simulink model "com_detect_red_circle"  (R2016b)
settings: Solver=VariableStepAuto  StartTime=0.0  StopTime=inf  RelTol=1e-3
values from neighbouring files (symbols this model uses):
  hmax = inrange.h_max_r    [computer_detectTrafficLight.m]    (also in getColorPX.m = h)
  hmin = inrange.h_min_r    [computer_detectTrafficLight.m]    (also in getColorPX.m = h)
  smax = inrange.s_max_r    [computer_detectTrafficLight.m]    (also in getColorPX.m = s)
  smin = inrange.s_min_r    [computer_detectTrafficLight.m]    (also in getColorPX.m = s)
  vmax = inrange.v_max_r    [computer_detectTrafficLight.m]    (also in getColorPX.m = v)
  vmin = inrange.v_min_r    [computer_detectTrafficLight.m]    (also in getColorPX.m = v)
undefined symbols (not defined in the file or in its folder): gray, Rec, SDTV, strel
libraries: etargetslib x15, dspnetwork x15, visionconversions x5, visiongeotforms x3, visionmorphops x2, visiontextngfix x1
settings Model: Creator=zeabus  LastModifiedBy=zeabus

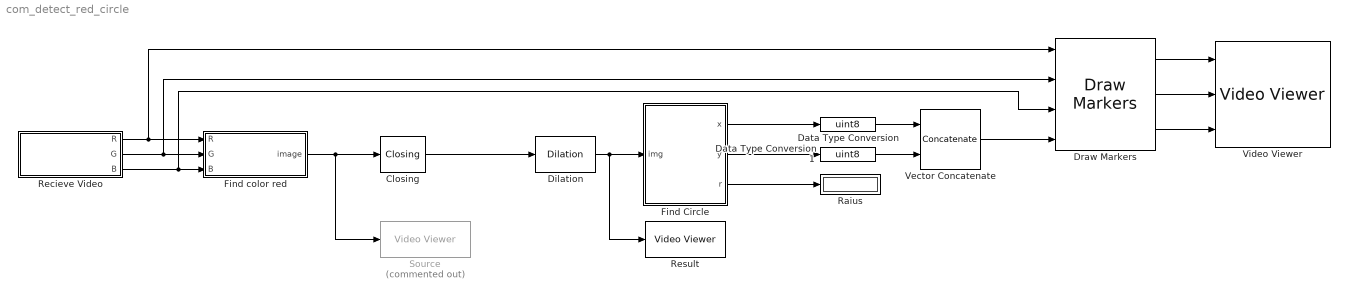
== system com_detect_red_circle ==
  Closing : visionmorphops/Closing  nhoodsrc=Specify via dialog  strel=strel('line', 10, 45)
  Data Type Conversion : DataTypeConversion  OutDataTypeStr=uint8
  Data Type Conversion1 : DataTypeConversion  OutDataTypeStr=uint8
  Dilation : visionmorphops/Dilation  nhoodsrc=Specify via dialog  strel=[40 40 40; 40 40 40; 40 40 40]
  Draw Markers : visiontextngfix/Draw Markers  shape=Circle  size=20  fill=on  fillClrSource=Specify via dialog  display=User-specified value  intensity=200  color=[255 255 0]  opacity=0.6  viewport=Entire image  antialiasing=off  inType=Obsolete  imagePorts=Separate color signals  prodOutputMode=Binary point scaling  prodOutputWordLength=32  prodOutputFracLength=14  memoryMode=Specify word length  memoryWordLength=16  memoryFracLength=14  roundingMode=Floor  overflowMode=off
  Find Circle : MATLAB Function  TreatAsAtomicUnit=on
  Find color red : Subsystem
  Raius : Display
  Recieve Video : Subsystem
  Result : VideoViewer  FigPos=[-15 1005 811 384]
  Source : VideoViewer  Commented=on  colormapValue=gray(256)  FigPos=[-22 597 811 384]
  Vector Concatenate : Concatenate  Mode=Multidimensional array
  Video Viewer : VideoViewer  imagePorts=separate color signals  FigPos=[1334 859 660 461]
  wires:
  Draw Markers/1 -> Video Viewer/1
  Draw Markers/2 -> Video Viewer/2
  Draw Markers/3 -> Video Viewer/3
  Find Circle/1(x) -> Data Type Conversion/1
  Find Circle/2(y) -> Data Type Conversion1/1
  Vector Concatenate/1 -> Draw Markers/4
  Data Type Conversion/1 -> Vector Concatenate/1
  Data Type Conversion1/1 -> Vector Concatenate/2
  Find color red/1(image) -> Source/1, Closing/1
  Dilation/1 -> Result/1, Find Circle/1(img)
  Find Circle/3(r) -> Raius/1
  Closing/1 -> Dilation/1
  Recieve Video/1(R) -> Draw Markers/1, Find color red/1(R)
  Recieve Video/2(G) -> Draw Markers/2, Find color red/2(G)
  Recieve Video/3(B) -> Draw Markers/3, Find color red/3(B)

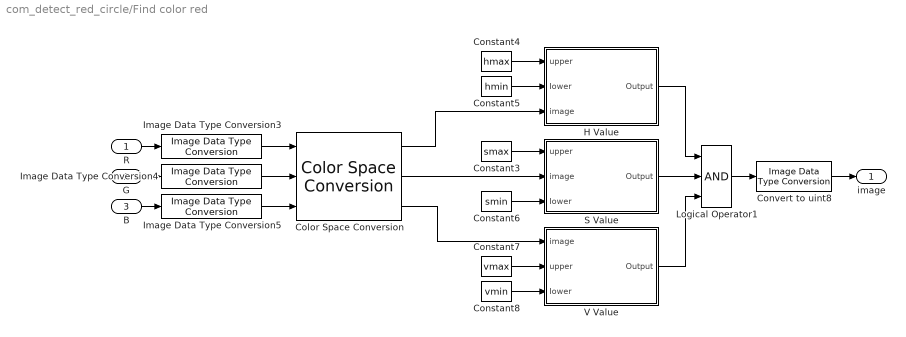
== system com_detect_red_circle/Find color red ==
  R : Inport
  G : Inport  Port=2
  B : Inport  Port=3
  Color Space Conversion : visionconversions/Color Space  Conversion  conversion=Obsolete  conversionActive=R'G'B' to HSV  wp_str=D65  rec=Rec. 601 (SDTV)  sys=1125/60/2:1  imagePorts=Separate color signals
  Constant3 : Constant  Value=smax
  Constant4 : Constant  Value=hmax
  Constant5 : Constant  Value=hmin
  Constant6 : Constant  Value=smin
  Constant7 : Constant  Value=vmax
  Constant8 : Constant  Value=vmin
  Convert to uint8 : visionconversions/Image Data Type Conversion  outDT=uint8  isSigned=on  wordLen=16  numFracBits=0
  H Value : Subsystem
  Image Data Type Conversion3 : visionconversions/Image Data Type Conversion  outDT=single  isSigned=on  wordLen=16  numFracBits=0
  Image Data Type Conversion4 : visionconversions/Image Data Type Conversion  outDT=single  isSigned=on  wordLen=16  numFracBits=0
  Image Data Type Conversion5 : visionconversions/Image Data Type Conversion  outDT=single  isSigned=on  wordLen=16  numFracBits=0
  Logical Operator1 : Logic  Inputs=3  AllPortsSameDT=off  OutDataTypeStr=boolean
  S Value : Subsystem
  V Value : Subsystem
  image : Outport
  wires:
  Color Space Conversion/1 -> H Value/3(image)
  Constant5/1 -> H Value/2(Iower)
  Color Space Conversion/2 -> S Value/2(image)
  Constant3/1 -> S Value/1(upper)
  Constant6/1 -> S Value/3(Iower)
  Color Space Conversion/3 -> V Value/1(image)
  Constant7/1 -> V Value/2(upper)
  Constant8/1 -> V Value/3(Iower)
  H Value/1(Output) -> Logical Operator1/1
  S Value/1(Output) -> Logical Operator1/2
  V Value/1(Output) -> Logical Operator1/3
  Image Data Type Conversion3/1 -> Color Space Conversion/1
  Image Data Type Conversion4/1 -> Color Space Conversion/2
  Image Data Type Conversion5/1 -> Color Space Conversion/3
  Logical Operator1/1 -> Convert to uint8/1
  R/1 -> Image Data Type Conversion3/1
  G/1 -> Image Data Type Conversion4/1
  B/1 -> Image Data Type Conversion5/1
  Constant4/1 -> H Value/1(upper)
  Convert to uint8/1 -> image/1

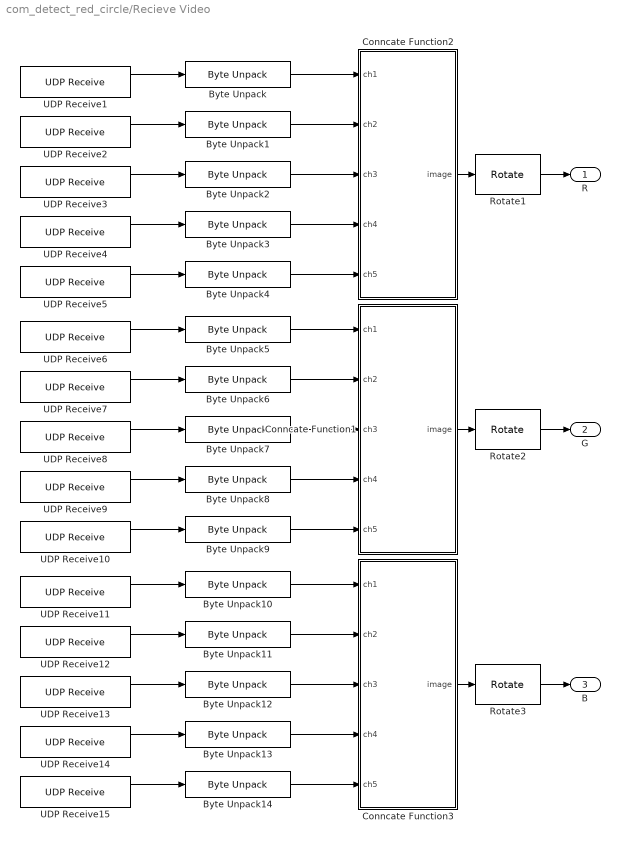
== system com_detect_red_circle/Recieve Video ==
  Byte Unpack{,1..14} (15 alike) : etargetslib/Byte Unpack  dimensions={[15360]}  datatypes={'uint8'}  byteAlign=1
  Conncate Function1 : MATLAB Function  TreatAsAtomicUnit=on
  Conncate Function2 : MATLAB Function  TreatAsAtomicUnit=on
  Conncate Function3 : MATLAB Function  TreatAsAtomicUnit=on
  Rotate1 : visiongeotforms/Rotate  outSizeR=Expanded to fit rotated input image  src_angle=Specify via dialog  unit_angle=Degrees  angle=-pi/2  maxAngle=pi  dispImage=Center  method=Table lookup  fillVal=0  interpMethod=Bilinear  prodOutputMode=Binary point scaling  prodOutputWordLength=32  prodOutputFracLength=10  roundingMode=Nearest  overflowMode=on
  Rotate2 : visiongeotforms/Rotate  outSizeR=Expanded to fit rotated input image  src_angle=Specify via dialog  unit_angle=Degrees  angle=-pi/2  maxAngle=pi  dispImage=Center  method=Table lookup  fillVal=0  interpMethod=Bilinear  prodOutputMode=Binary point scaling  prodOutputWordLength=32  prodOutputFracLength=10  roundingMode=Nearest  overflowMode=on
  Rotate3 : visiongeotforms/Rotate  outSizeR=Expanded to fit rotated input image  src_angle=Specify via dialog  unit_angle=Degrees  angle=-pi/2  maxAngle=pi  dispImage=Center  method=Table lookup  fillVal=0  interpMethod=Bilinear  prodOutputMode=Binary point scaling  prodOutputWordLength=32  prodOutputFracLength=10  roundingMode=Nearest  overflowMode=on
  UDP Receive1 : dspnetwork/UDP Receive  localURL='0.0.0.0'  localPort=30000  remoteURL='0.0.0.0'  remotePort=-1  recvBufferSize=61500  dims=15360  signalDatatype=uint8  isVarSize=off  showBlockingTime=on  blockingTime=0.01  sampletime=0.01  blockPlatform=HOST
  UDP Receive10 : dspnetwork/UDP Receive  localURL='0.0.0.0'  localPort=30009  remoteURL='0.0.0.0'  remotePort=-1  recvBufferSize=61500  dims=15360  signalDatatype=uint8  isVarSize=off  showBlockingTime=on  blockingTime=0.03  sampletime=0.03  blockPlatform=HOST
  UDP Receive11 : dspnetwork/UDP Receive  localURL='0.0.0.0'  localPort=30010  remoteURL='0.0.0.0'  remotePort=-1  recvBufferSize=61500  dims=15360  signalDatatype=uint8  isVarSize=off  showBlockingTime=on  blockingTime=0.03  sampletime=0.03  blockPlatform=HOST
  UDP Receive12 : dspnetwork/UDP Receive  localURL='0.0.0.0'  localPort=30011  remoteURL='0.0.0.0'  remotePort=-1  recvBufferSize=61500  dims=15360  signalDatatype=uint8  isVarSize=off  showBlockingTime=on  blockingTime=0.03  sampletime=0.03  blockPlatform=HOST
  UDP Receive13 : dspnetwork/UDP Receive  localURL='0.0.0.0'  localPort=30012  remoteURL='0.0.0.0'  remotePort=-1  recvBufferSize=61500  dims=15360  signalDatatype=uint8  isVarSize=off  showBlockingTime=on  blockingTime=0.03  sampletime=0.03  blockPlatform=HOST
  UDP Receive14 : dspnetwork/UDP Receive  localURL='0.0.0.0'  localPort=30013  remoteURL='0.0.0.0'  remotePort=-1  recvBufferSize=61500  dims=15360  signalDatatype=uint8  isVarSize=off  showBlockingTime=on  blockingTime=0.03  sampletime=0.03  blockPlatform=HOST
  UDP Receive15 : dspnetwork/UDP Receive  localURL='0.0.0.0'  localPort=30014  remoteURL='0.0.0.0'  remotePort=-1  recvBufferSize=61500  dims=15360  signalDatatype=uint8  isVarSize=off  showBlockingTime=on  blockingTime=0.03  sampletime=0.03  blockPlatform=HOST
  UDP Receive2 : dspnetwork/UDP Receive  localURL='0.0.0.0'  localPort=30001  remoteURL='0.0.0.0'  remotePort=-1  recvBufferSize=61500  dims=15360  signalDatatype=uint8  isVarSize=off  showBlockingTime=on  blockingTime=0.01  sampletime=0.01  blockPlatform=HOST
  UDP Receive3 : dspnetwork/UDP Receive  localURL='0.0.0.0'  localPort=30002  remoteURL='0.0.0.0'  remotePort=-1  recvBufferSize=61500  dims=15360  signalDatatype=uint8  isVarSize=off  showBlockingTime=on  blockingTime=0.01  sampletime=0.01  blockPlatform=HOST
  UDP Receive4 : dspnetwork/UDP Receive  localURL='0.0.0.0'  localPort=30003  remoteURL='0.0.0.0'  remotePort=-1  recvBufferSize=61500  dims=15360  signalDatatype=uint8  isVarSize=off  showBlockingTime=on  blockingTime=0.01  sampletime=0.01  blockPlatform=HOST
  UDP Receive5 : dspnetwork/UDP Receive  localURL='0.0.0.0'  localPort=30004  remoteURL='0.0.0.0'  remotePort=-1  recvBufferSize=61500  dims=15360  signalDatatype=uint8  isVarSize=off  showBlockingTime=on  blockingTime=0.01  sampletime=0.01  blockPlatform=HOST
  UDP Receive6 : dspnetwork/UDP Receive  localURL='0.0.0.0'  localPort=30005  remoteURL='0.0.0.0'  remotePort=-1  recvBufferSize=61500  dims=15360  signalDatatype=uint8  isVarSize=off  showBlockingTime=on  blockingTime=0.03  sampletime=0.03  blockPlatform=HOST
  UDP Receive7 : dspnetwork/UDP Receive  localURL='0.0.0.0'  localPort=30006  remoteURL='0.0.0.0'  remotePort=-1  recvBufferSize=61500  dims=15360  signalDatatype=uint8  isVarSize=off  showBlockingTime=on  blockingTime=0.03  sampletime=0.03  blockPlatform=HOST
  UDP Receive8 : dspnetwork/UDP Receive  localURL='0.0.0.0'  localPort=30007  remoteURL='0.0.0.0'  remotePort=-1  recvBufferSize=61500  dims=15360  signalDatatype=uint8  isVarSize=off  showBlockingTime=on  blockingTime=0.03  sampletime=0.03  blockPlatform=HOST
  UDP Receive9 : dspnetwork/UDP Receive  localURL='0.0.0.0'  localPort=30008  remoteURL='0.0.0.0'  remotePort=-1  recvBufferSize=61500  dims=15360  signalDatatype=uint8  isVarSize=off  showBlockingTime=on  blockingTime=0.03  sampletime=0.03  blockPlatform=HOST
  R : Outport
  G : Outport  Port=2
  B : Outport  Port=3
  wires:
  UDP Receive1/1 -> Byte Unpack/1
  UDP Receive2/1 -> Byte Unpack1/1
  UDP Receive3/1 -> Byte Unpack2/1
  UDP Receive4/1 -> Byte Unpack3/1
  UDP Receive5/1 -> Byte Unpack4/1
  Byte Unpack3/1 -> Conncate Function2/4(ch4)
  Byte Unpack4/1 -> Conncate Function2/5(ch5)
  Byte Unpack2/1 -> Conncate Function2/3(ch3)
  Byte Unpack1/1 -> Conncate Function2/2(ch2)
  Byte Unpack/1 -> Conncate Function2/1(ch1)
  UDP Receive6/1 -> Byte Unpack5/1
  UDP Receive7/1 -> Byte Unpack6/1
  UDP Receive8/1 -> Byte Unpack7/1
  UDP Receive9/1 -> Byte Unpack8/1
  UDP Receive10/1 -> Byte Unpack9/1
  Byte Unpack8/1 -> Conncate Function1/4(ch4)
  Byte Unpack9/1 -> Conncate Function1/5(ch5)
  Byte Unpack7/1 -> Conncate Function1/3(ch3)
  Byte Unpack6/1 -> Conncate Function1/2(ch2)
  Byte Unpack5/1 -> Conncate Function1/1(ch1)
  UDP Receive11/1 -> Byte Unpack10/1
  UDP Receive12/1 -> Byte Unpack11/1
  UDP Receive13/1 -> Byte Unpack12/1
  UDP Receive14/1 -> Byte Unpack13/1
  UDP Receive15/1 -> Byte Unpack14/1
  Byte Unpack13/1 -> Conncate Function3/4(ch4)
  Byte Unpack14/1 -> Conncate Function3/5(ch5)
  Byte Unpack12/1 -> Conncate Function3/3(ch3)
  Byte Unpack11/1 -> Conncate Function3/2(ch2)
  Byte Unpack10/1 -> Conncate Function3/1(ch1)
  Conncate Function2/1(image) -> Rotate1/1
  Conncate Function1/1(image) -> Rotate2/1
  Conncate Function3/1(image) -> Rotate3/1
  Rotate1/1 -> R/1
  Rotate2/1 -> G/1
  Rotate3/1 -> B/1

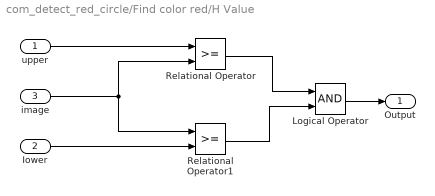
== system com_detect_red_circle/Find color red/H Value ==
  upper : Inport
  Iower : Inport  Port=2
  image : Inport  Port=3
  Logical Operator : Logic  AllPortsSameDT=off  OutDataTypeStr=boolean
  Relational Operator : RelationalOperator  OutDataTypeStr=boolean  RndMeth=Simplest
  Relational Operator1 : RelationalOperator  OutDataTypeStr=boolean  RndMeth=Simplest
  Output : Outport
  wires:
  upper/1 -> Relational Operator/1
  Iower/1 -> Relational Operator1/2
  image/1 -> Relational Operator/2, Relational Operator1/1
  Relational Operator/1 -> Logical Operator/1
  Relational Operator1/1 -> Logical Operator/2
  Logical Operator/1 -> Output/1

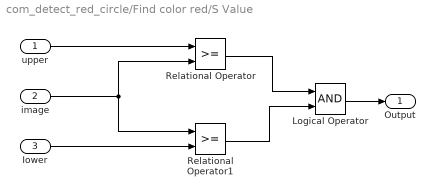
== system com_detect_red_circle/Find color red/S Value ==
  upper : Inport
  image : Inport  Port=2
  Iower : Inport  Port=3
  Logical Operator : Logic  AllPortsSameDT=off  OutDataTypeStr=boolean
  Relational Operator : RelationalOperator  OutDataTypeStr=boolean  RndMeth=Simplest
  Relational Operator1 : RelationalOperator  OutDataTypeStr=boolean  RndMeth=Simplest
  Output : Outport
  wires:
  upper/1 -> Relational Operator/1
  Iower/1 -> Relational Operator1/2
  image/1 -> Relational Operator/2, Relational Operator1/1
  Relational Operator/1 -> Logical Operator/1
  Relational Operator1/1 -> Logical Operator/2
  Logical Operator/1 -> Output/1

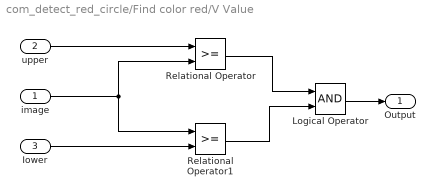
== system com_detect_red_circle/Find color red/V Value ==
  image : Inport
  upper : Inport  Port=2
  Iower : Inport  Port=3
  Logical Operator : Logic  AllPortsSameDT=off  OutDataTypeStr=boolean
  Relational Operator : RelationalOperator  OutDataTypeStr=boolean  RndMeth=Simplest
  Relational Operator1 : RelationalOperator  OutDataTypeStr=boolean  RndMeth=Simplest
  Output : Outport
  wires:
  upper/1 -> Relational Operator/1
  Iower/1 -> Relational Operator1/2
  image/1 -> Relational Operator/2, Relational Operator1/1
  Relational Operator/1 -> Logical Operator/1
  Relational Operator1/1 -> Logical Operator/2
  Logical Operator/1 -> Output/1

== matlab function com_detect_red_circle/Recieve Video/Conncate Function2 ==
  data: ch1 input; ch2 input; ch3 input; ch4 input; ch5 input uint8; image output
function image  = concatenation(ch1,ch2,ch3,ch4,ch5)
maxcol = 48;
height = 320;
width = 240;
ch1 = reshape(ch1,height,maxcol);
ch2 = reshape(ch2,height,maxcol);
ch3 = reshape(ch3,height,maxcol);
ch4 = reshape(ch4,height,maxcol);
ch5 = reshape(ch5,height,maxcol);
image = [ch1,ch2,ch3,ch4,ch5];
image = reshape(image,height,width);

== matlab function com_detect_red_circle/Recieve Video/Conncate Function1 ==
  data: ch1 input; ch2 input; ch3 input; ch4 input; ch5 input uint8; image output
function image  = concatenation(ch1,ch2,ch3,ch4,ch5)
maxcol = 48;
height = 320;
width = 240;
ch1 = reshape(ch1,height,maxcol);
ch2 = reshape(ch2,height,maxcol);
ch3 = reshape(ch3,height,maxcol);
ch4 = reshape(ch4,height,maxcol);
ch5 = reshape(ch5,height,maxcol);
image = [ch1,ch2,ch3,ch4,ch5];
image = reshape(image,height,width);

== matlab function com_detect_red_circle/Recieve Video/Conncate Function3 ==
  data: ch1 input; ch2 input; ch3 input; ch4 input; ch5 input uint8; image output
function image  = concatenation(ch1,ch2,ch3,ch4,ch5)
maxcol = 48;
height = 320;
width = 240;
ch1 = reshape(ch1,height,maxcol);
ch2 = reshape(ch2,height,maxcol);
ch3 = reshape(ch3,height,maxcol);
ch4 = reshape(ch4,height,maxcol);
ch5 = reshape(ch5,height,maxcol);
image = [ch1,ch2,ch3,ch4,ch5];
image = reshape(image,height,width);

== matlab function com_detect_red_circle/Find Circle ==
  data: img input; x output; y output; r output
% Author : Supakit Kriangkhajorn,'Sensitivity',0.7
% Follow me : skconan

function [x,y,r]= findcircle(img)
    coder.extrinsic('imfindcircles'); 
    coder.extrinsic('isempty');
    coder.extrinsic('sortrows');
    coder.extrinsic('size');
    coder.extrinsic('graythresh');
    x = 150;
    y = 150;
    r = 0;
    centerMax = [0,0];
    cols = 0;
    status = 0;
    level = graythresh(img)
    [centers, radius, metric] = imfindcircles(img,[10 90],'Sensitivity',0.97,...
                                'Method','twostage','EdgeThreshold',level,...
                                'ObjectPolarity','bright');
    circles = [centers, radius, metric];
    check = ~isempty(circles);
    if check
        status = 1;
        circles = sortrows(circles,3);
        [rows,cols] = size(circles);
        centerMax = circles(rows,1:2);
        r = circles(rows,3); 
    end
         
x = round(centerMax(1));
y = round(centerMax(2));
